simulink model "Particulas"  (R2020b)
settings: Solver=ode45  StartTime=0.0  StopTime=200  FixedStep=1e-7  RelTol=1e-4  AbsTol=1e-4  EnableMultiTasking=on
settings Model: PacingRate=112  Creator=André  LastModifiedBy=Andre
settings SolverCC: AutoScaleAbsTol=off  ConsecutiveZCsStepRelTol=100*128*eps  ShapePreserveControl=EnableAll  ZeroCrossControl=EnableAll  AutoInsertRateTranBlk=on
settings DataIOCC: LimitDataPoints=on  SaveFormat=Array  SignalLoggingSaveFormat=ModelDataLogs  ReturnWorkspaceOutputs=off
settings OptimizationCC: ExpressionDepthLimit=2147483647  LifeSpan=inf
settings DebuggingCC: UnderspecifiedInitializationDetection=Classic  MergeDetectMultiDrivingBlocksExec=none  SolverPrmCheckMsg=warning  FcnCallInpInsideContextMsg=warning  StateNameClashWarn=warning  SFUnexpectedBacktrackingDiag=warning  SFNoUnconditionalDefaultTransitionDiag=warning  SFExecutionAtInitializationDiag=none  ArithmeticOperatorsInVariantConditions=warning
settings HardwareCC: ProdBitPerPointer=32  ProdBitPerSizeT=32  ProdBitPerPtrDiffT=32  ProdLargestAtomicFloat=None  ProdIntDivRoundTo=Undefined  ProdEndianess=Unspecified  ProdWordSize=32  ProdHWDeviceType=32-bit Generic
settings ModelReferenceCC: PropagateSignalLabelsOutOfModel=off
settings SFSimCC: SimUseLocalCustomCode=off  SimParseCustomCode=off  CustomCodeUndefinedFunction=UseInterfaceOnly
settings RTWCC: RTWUseLocalCustomCode=off
settings CodeAppCC: StateflowObjectComments=on
settings GRTTargetCC: TargetLangStandard=C89/C90 (ANSI)  CombineOutputUpdateFcns=off  GRTInterface=on
settings ConfigComp: CovMetricSettings=dw  CovSaveCumulativeToWorkspaceVar=on  CovSaveSingleToWorkspaceVar=on  CovExternalEMLEnable=off

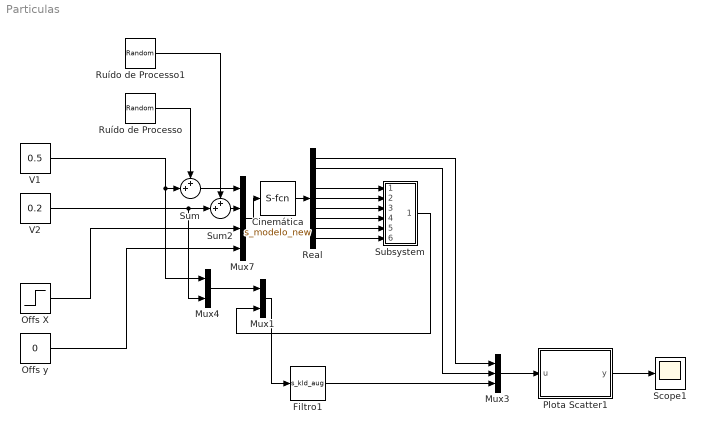
== system Particulas ==
  Cinemática : S-Function  FunctionName=s_modelo_new  Parameters=[1 2 pi/6]  SFunctionDeploymentMode=off  EnableBusSupport=off
  Filtro1 : S-Function  FunctionName=s_kld_aug  Parameters=[0 0 0]  SFunctionDeploymentMode=off  EnableBusSupport=off
  Mux1 : Mux  Inputs=2
  Mux3 : Mux  Inputs=3
  Mux4 : Mux  Inputs=2
  Mux7 : Mux
  Offs X : Step  Time=10  After=5  SampleTime=0
  Offs y : Constant  Value=0
  Plota Scatter1 : MATLAB Function  TreatAsAtomicUnit=on
  Real : Demux  Outputs=9
  Ruído de Processo : RandomNumber  Variance=0.1  SampleTime=0.1
  Ruído de Processo1 : RandomNumber  Variance=0.1  SampleTime=0.1
  Scope1 : Scope
  Subsystem : Subsystem
  Sum : Sum  Inputs=++|
  Sum2 : Sum  Inputs=++|
  V1 : Constant  Value=0.5
  V2 : Constant  Value=0.2
  wires:
  Mux1/1 -> Filtro1/1
  Ruído de Processo/1 -> Sum/1
  Mux7/1 -> Cinemática/1
  Sum2/1 -> Mux7/2
  V1/1 -> Mux4/1, Sum/2
  Sum/1 -> Mux7/1
  Mux4/1 -> Mux1/1
  Cinemática/1 -> Real/1
  V2/1 -> Mux4/2, Sum2/2
  Ruído de Processo1/1 -> Sum2/1
  Subsystem/1(Out1) -> Mux1/2
  Real/4 -> Subsystem/1(In1)
  Real/5 -> Subsystem/2(In2)
  Real/6 -> Subsystem/3(In3)
  Real/7 -> Subsystem/4(In4)
  Real/8 -> Subsystem/5(In5)
  Real/9 -> Subsystem/6(In6)
  Real/1 -> Mux3/1
  Real/2 -> Mux3/2
  Offs X/1 -> Mux7/3
  Offs y/1 -> Mux7/4
  Plota Scatter1/1(y) -> Scope1/1
  Mux3/1 -> Plota Scatter1/1(u)
  Filtro1/1 -> Mux3/3

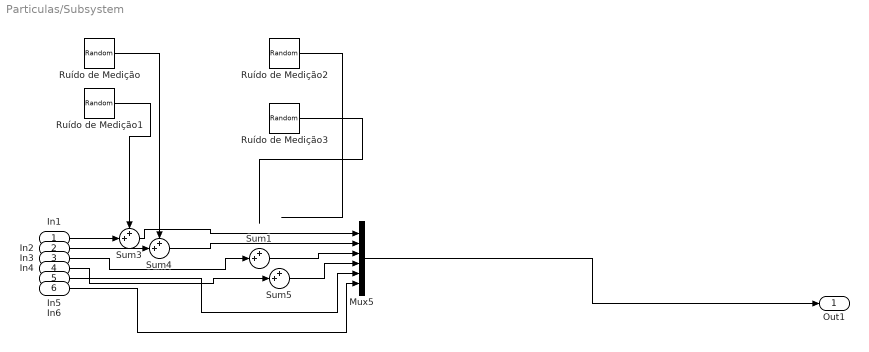
== system Particulas/Subsystem ==
  In1 : Inport
  In2 : Inport  Port=2
  In3 : Inport  Port=3
  In4 : Inport  Port=4
  In5 : Inport  Port=5
  In6 : Inport  Port=6
  Mux5 : Mux  Inputs=6
  Ruído de Medição{,1..3} (4 alike) : RandomNumber  Variance=0.1  SampleTime=0.01
  Sum{1,3..5} (4 alike) : Sum  Inputs=++|
  Out1 : Outport
  wires:
  Sum3/1 -> Mux5/1
  Ruído de Medição3/1 -> ?
  Ruído de Medição2/1 -> ?
  In2/1 -> Sum4/2
  Mux5/1 -> Out1/1
  Sum5/1 -> Mux5/4
  Ruído de Medição/1 -> Sum4/1
  Sum1/1 -> Mux5/3
  Sum4/1 -> Mux5/2
  Ruído de Medição1/1 -> Sum3/1
  In4/1 -> Sum5/2
  In1/1 -> Sum3/2
  In6/1 -> Mux5/6
  In3/1 -> Sum1/2
  In5/1 -> Mux5/5

== matlab function Particulas/Plota Scatter1 ==
  data: u input; y output
function  y=fcn(u)
     n_Particulas = u(3);  
     marker = [0 0; 5 5]; % Positions of markers
     n_estados = n_Particulas*3;
     %
     y=u(3:4);
     u = u([1:2,5:end]);
     %
     x = u(1:2);
     particulas = u(3:(2+n_estados));
     
     coder.extrinsic('scatter')
     
     
      xP = reshape(particulas,3,[]);
      x_ = mean(xP, 2);
      %x_ = u(3+n_estados:5+n_estados);
      %figure(1);
      scatter(xP(1,:),xP(2,:), 'k.');
      axis( [-10 10 -10 10]);
      hold on;
      text(0,0,string(n_Particulas));
      %figure(1);
      scatter(x_(1),x_(2),'bo');
      scatter(marker(:,1),marker(:,2), 'gs');
      scatter(x(1),x(2), 'r*');
      hold off;
     % insert additional code as needed to turn on grid, setup axis limits, etc.

  %%%%%%%%%
%y = u;
